simulink model "lineFollowerModel"  (R2020a)
settings: Solver=ode4  StartTime=0.0  StopTime=50  FixedStep=0.0001  RelTol=1e-3
values from neighbouring files (symbols this model uses):
  b = -0.05    [define_constants.m]
  cRoll = 0.1    [define_constants.m]
  g = 9.81    [define_constants.m]
  I_T = 0.1    [define_constants.m]
  I_yy = 5.0000e-05    (= 5e-05)    [define_constants.m]
  K = 0.0089    [define_constants.m]
  L = 2.3E-2    (= 0.023)    [define_constants.m]
  m_T = 1 * mass_scale    [define_constants.m]
  N = 50    [define_constants.m]
  R = 2.2    [define_constants.m]
  row1 = 0.1    [define_constants.m]
  row2 = row1*wheel_ratio_scale    [define_constants.m]
  sX_FL = 0.05    [define_constants.m]
  sX_FR = 0.05    [define_constants.m]
  sX_L = 0.05    [define_constants.m]
  sX_R = 0.05    [define_constants.m]
  sY_FL = 0.060    (= 0.06)    [define_constants.m]
  sY_FR = -0.060    (= -0.06)    [define_constants.m]
  sY_L = 0.03    [define_constants.m]
  sY_R = -0.03    [define_constants.m]
  Vmax = 12    [define_constants.m]
  W = line_width/2    [define_constants.m]
libraries: simulink x4
settings Model: Creator=Amir  LastModifiedBy=aekha
settings SFSimCC: CustomCodeUndefinedFunction=UseInterfaceOnly

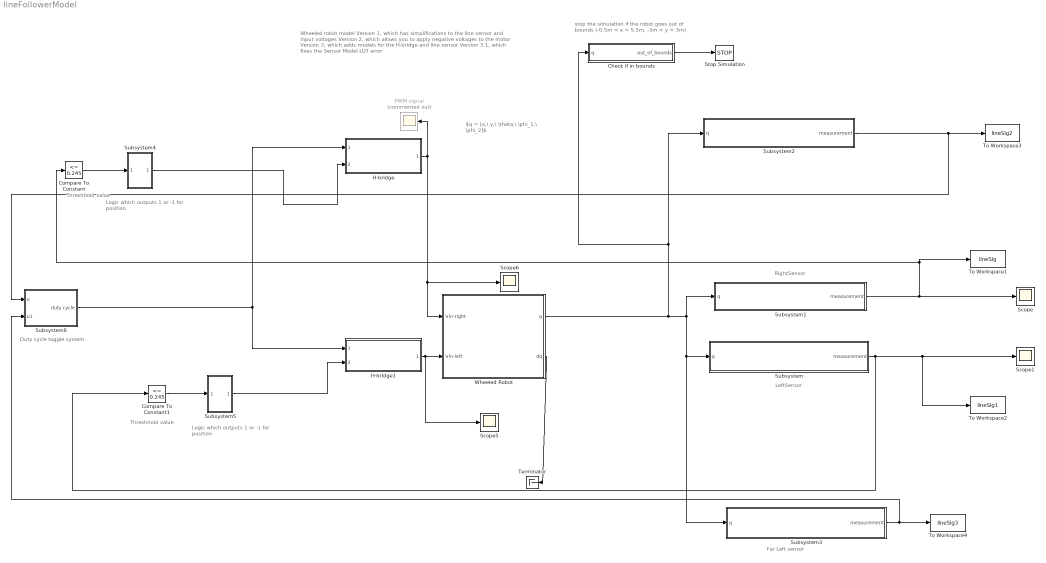
== system lineFollowerModel ==
  note: Threshhold value
  note: Duty cycle toggle system
  note: Far Left sensor
  note: Logic which outputs 1 or -1
      | for position
  note: LeftSensor
  note: RightSensor
  note: stop the simulation if the robot goes out of bounds (-0.5m < x < 5.5m, -3m < y < 3m)
  note: Wheeled robot model
      | Version 1, which has simplifications to the line sensor and input voltages
      | Version 2, which allows you to apply negative voltages to the motor
      | Version 3, which adds models for the H-bridge and line sensor
      | Version 3.1, which fixes the Sensor Model LUT error
  note: $q = [x,\ y,\ \theta,\ \phi_1,\ \phi_2]$
  note: Logic which outputs 1 or -1
      | for position
  note: Threshhold value
  Check if in bounds : MATLAB Function  TreatAsAtomicUnit=on
  Compare To Constant : simulink/Logic and Bit Operations/Compare To Constant  relop=<=  const=0.245  OutDataTypeStr=boolean
  Compare To Constant1 : simulink/Logic and Bit Operations/Compare To Constant  relop=<=  const=0.245  OutDataTypeStr=boolean
  H-bridge : Subsystem  ReferencedSubsystem=H_bridge
  H-bridge1 : Subsystem  ReferencedSubsystem=H_bridge
  PWM signal : Scope  Commented=on
  Scope{,1,5..6} (4 alike) : Scope
  Stop Simulation : Stop
  Subsystem : Subsystem
  Subsystem1 : Subsystem
  Subsystem2 : Subsystem
  Subsystem3 : Subsystem
  Subsystem4 : Subsystem
  Subsystem5 : Subsystem
  Subsystem6 : Subsystem
  Terminator : Terminator
  To Workspace1 : ToWorkspace  VariableName=lineSig  SampleTime=-1
  To Workspace2 : ToWorkspace  VariableName=lineSig1  SampleTime=-1
  To Workspace3 : ToWorkspace  VariableName=lineSig2  SampleTime=-1
  To Workspace4 : ToWorkspace  VariableName=lineSig3  SampleTime=-1
  Wheeled Robot : Subsystem
  wires:
  H-bridge/1 -> Scope6/1, Wheeled Robot/1(Vin-right), PWM signal/1
  H-bridge1/1 -> Scope5/1, Wheeled Robot/2(Vin-left)
  Wheeled Robot/2(dq) -> Terminator/1
  Check if in bounds/1(out_of_bounds) -> Stop Simulation/1
  Subsystem/1(measurement) -> Compare To Constant1/1, To Workspace2/1, Scope1/1
  Subsystem1/1(measurement) -> To Workspace1/1, Compare To Constant/1, Scope/1
  Subsystem3/1(measurement) -> Subsystem6/2(u1), To Workspace4/1
  Subsystem2/1(measurement) -> Subsystem6/1(u), To Workspace3/1
  Subsystem4/1(direction) -> H-bridge/2
  Wheeled Robot/1(q) -> Subsystem/1(q), Subsystem3/1(q), Subsystem1/1(q), Check if in bounds/1(q), Subsystem2/1(q)
  Subsystem5/1(direction) -> H-bridge1/2
  Compare To Constant/1 -> Subsystem4/1(In1)
  Compare To Constant1/1 -> Subsystem5/1(In1)
  Subsystem6/1(duty cycle) -> H-bridge1/1, H-bridge/1

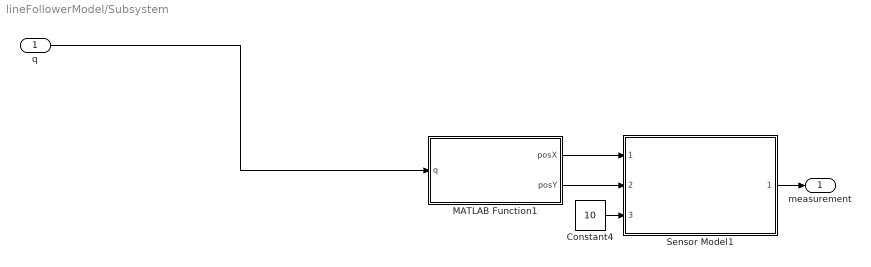
== system lineFollowerModel/Subsystem ==
  q : Inport
  Constant4 : Constant  Value=10
  MATLAB Function1 : MATLAB Function  TreatAsAtomicUnit=on
  Sensor Model1 : Subsystem  ReferencedSubsystem=Sensor_Model
  measurement : Outport
  wires:
  Constant4/1 -> Sensor Model1/3
  MATLAB Function1/2(posY) -> Sensor Model1/2
  Sensor Model1/1 -> measurement/1
  MATLAB Function1/1(posX) -> Sensor Model1/1
  q/1 -> MATLAB Function1/1(q)

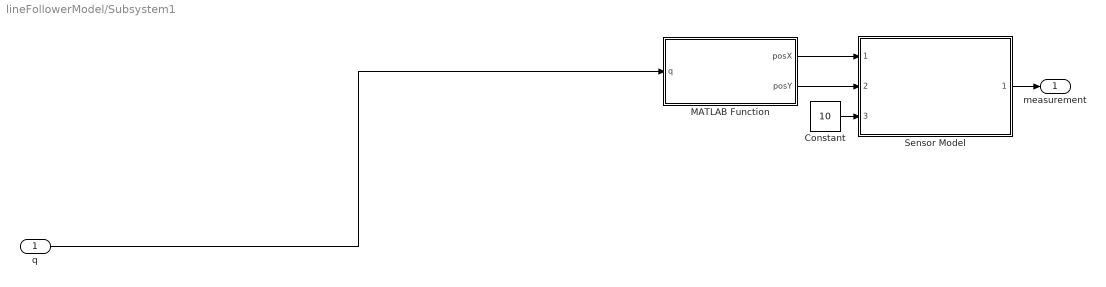
== system lineFollowerModel/Subsystem1 ==
  q : Inport
  Constant : Constant  Value=10
  MATLAB Function : MATLAB Function  TreatAsAtomicUnit=on
  Sensor Model : Subsystem  ReferencedSubsystem=Sensor_Model
  measurement : Outport
  wires:
  Constant/1 -> Sensor Model/3
  MATLAB Function/1(posX) -> Sensor Model/1
  q/1 -> MATLAB Function/1(q)
  Sensor Model/1 -> measurement/1
  MATLAB Function/2(posY) -> Sensor Model/2

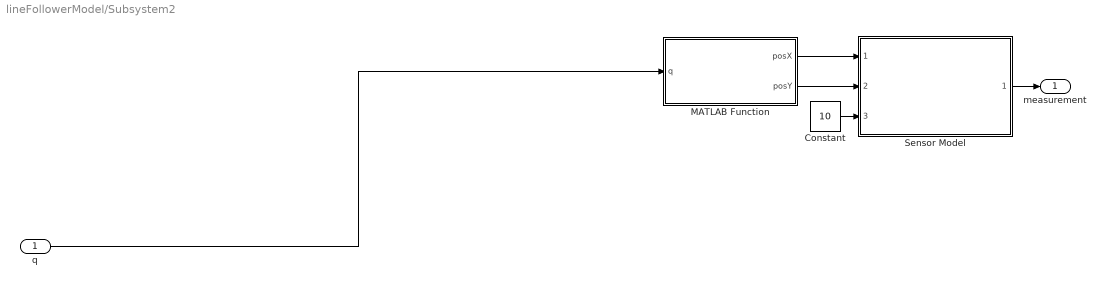
== system lineFollowerModel/Subsystem2 ==
  q : Inport
  Constant : Constant  Value=10
  MATLAB Function : MATLAB Function  TreatAsAtomicUnit=on
  Sensor Model : Subsystem  ReferencedSubsystem=Sensor_Model
  measurement : Outport
  wires:
  Constant/1 -> Sensor Model/3
  MATLAB Function/1(posX) -> Sensor Model/1
  q/1 -> MATLAB Function/1(q)
  Sensor Model/1 -> measurement/1
  MATLAB Function/2(posY) -> Sensor Model/2

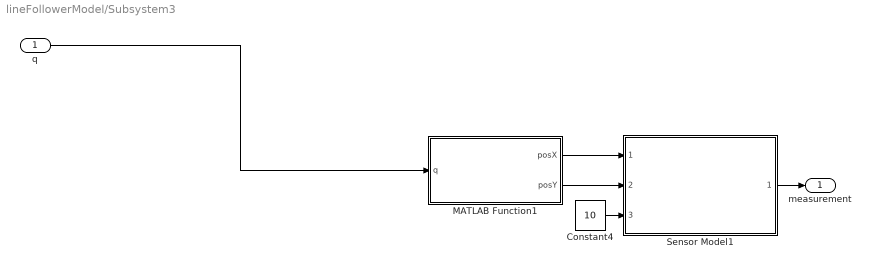
== system lineFollowerModel/Subsystem3 ==
  q : Inport
  Constant4 : Constant  Value=10
  MATLAB Function1 : MATLAB Function  TreatAsAtomicUnit=on
  Sensor Model1 : Subsystem  ReferencedSubsystem=Sensor_Model
  measurement : Outport
  wires:
  Constant4/1 -> Sensor Model1/3
  MATLAB Function1/2(posY) -> Sensor Model1/2
  Sensor Model1/1 -> measurement/1
  MATLAB Function1/1(posX) -> Sensor Model1/1
  q/1 -> MATLAB Function1/1(q)

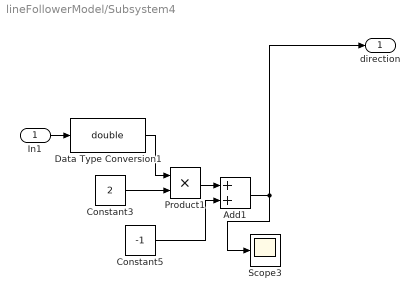
== system lineFollowerModel/Subsystem4 ==
  In1 : Inport
  Add1 : Sum
  Constant3 : Constant  Value=2
  Constant5 : Constant  Value=-1
  Data Type Conversion1 : DataTypeConversion  OutDataTypeStr=double
  Product1 : Product
  Scope3 : Scope
  direction : Outport
  wires:
  Data Type Conversion1/1 -> Product1/1
  Add1/1 -> direction/1, Scope3/1
  Constant5/1 -> Add1/2
  Product1/1 -> Add1/1
  In1/1 -> Data Type Conversion1/1
  Constant3/1 -> Product1/2

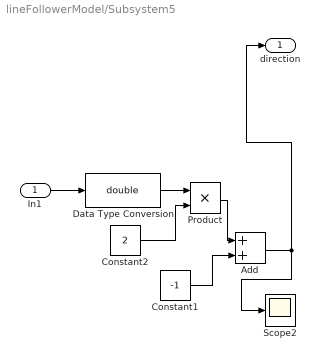
== system lineFollowerModel/Subsystem5 ==
  In1 : Inport
  Add : Sum
  Constant1 : Constant  Value=-1
  Constant2 : Constant  Value=2
  Data Type Conversion : DataTypeConversion  OutDataTypeStr=double
  Product : Product
  Scope2 : Scope
  direction : Outport
  wires:
  Constant2/1 -> Product/2
  Product/1 -> Add/1
  Add/1 -> direction/1, Scope2/1
  In1/1 -> Data Type Conversion/1
  Constant1/1 -> Add/2
  Data Type Conversion/1 -> Product/1

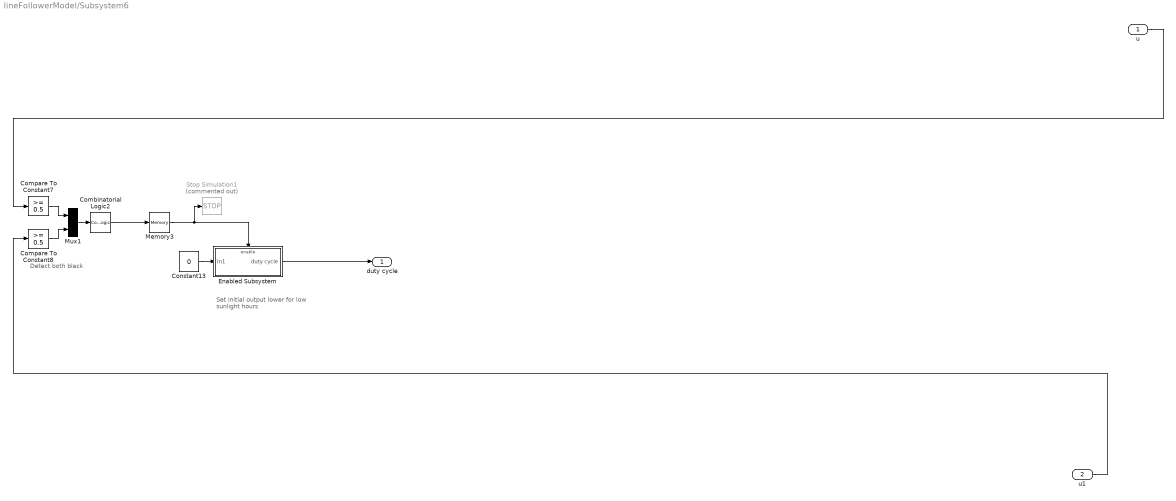
== system lineFollowerModel/Subsystem6 ==
  note: Detect both black
  note: Set initial output
      |  lower for low sunlight hours
  u : Inport
  u1 : Inport  Port=2
  Combinatorial Logic2 : CombinatorialLogic  TruthTable=[0;0;0;1]
  Compare To Constant7 : simulink/Logic and Bit Operations/Compare To Constant  relop=>=  const=0.5  OutDataTypeStr=boolean
  Compare To Constant8 : simulink/Logic and Bit Operations/Compare To Constant  relop=>=  const=0.5  OutDataTypeStr=boolean
  Constant13 : Constant  Value=0
  Enabled Subsystem : Subsystem  TreatAsAtomicUnit=on
  Memory3 : Memory
  Mux1 : Mux  Inputs=2
  Stop Simulation1 : Stop  Commented=on
  duty cycle : Outport
  wires:
  Compare To Constant8/1 -> Mux1/2
  Combinatorial Logic2/1 -> Memory3/1
  Memory3/1 -> Stop Simulation1/1, Enabled Subsystem/Enable
  Compare To Constant7/1 -> Mux1/1
  Mux1/1 -> Combinatorial Logic2/1
  Constant13/1 -> Enabled Subsystem/1(In1)
  u/1 -> Compare To Constant7/1
  Enabled Subsystem/1(duty cycle) -> duty cycle/1
  u1/1 -> Compare To Constant8/1

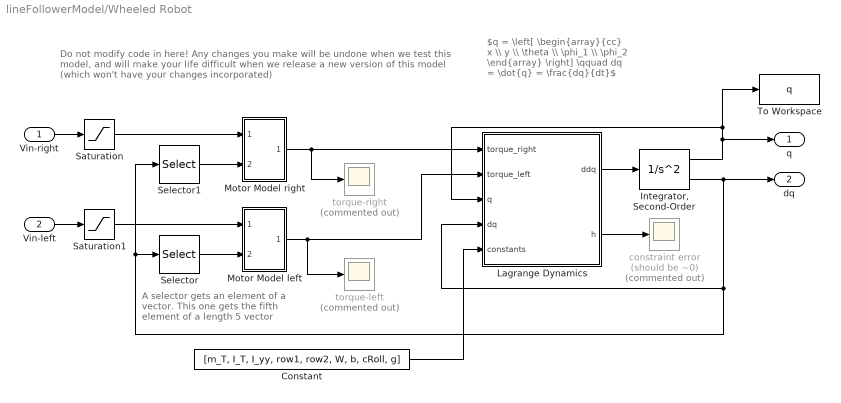
== system lineFollowerModel/Wheeled Robot ==
  note: A selector gets an element of a vector. This one gets the fifth element of a length 5 vector
  note: Do not modify code in here! Any changes you make will be undone when we test this model, and will make your life difficult when we release a new version of this model (which won't have your changes incorporated)
  note: $q = \left[ \begin{array}{cc} x \\ y \\ \theta \\ \phi_1 \\ \phi_2 \end{array} \right] \qquad dq = \dot{q} = \frac{dq}{dt}$
  Vin-right : Inport
  Vin-left : Inport  Port=2
  Constant : Constant  Value=[m_T, I_T, I_yy, row1, row2, W, b, cRoll, g]
  "Integrator, Second-Order" : SecondOrderIntegrator  ICX=[0 0 0 0 0]  ICDXDT=[0 0 0 0 0]
  Lagrange Dynamics : MATLAB Function  TreatAsAtomicUnit=on
  "Motor Model left " : Subsystem
  Motor Model right : Subsystem
  Saturation : Saturate  UpperLimit=Vmax  LowerLimit=-Vmax
  Saturation1 : Saturate  UpperLimit=Vmax  LowerLimit=-Vmax
  Selector : Selector  InputPortWidth=5  IndexOptions=Index vector (dialog)  Indices=[5]  OutputSizes=1
  Selector1 : Selector  InputPortWidth=5  IndexOptions=Index vector (dialog)  Indices=[4]  OutputSizes=1
  To Workspace : ToWorkspace  VariableName=q  SampleTime=0.01
  constraint error (should be ~0) : Scope  Commented=on
  torque-left : Scope  Commented=on
  torque-right : Scope  Commented=on
  q : Outport
  dq : Outport  Port=2
  wires:
  Selector/1 -> "Motor Model left "/2(Omega)
  Selector1/1 -> Motor Model right/2(Omega)
  Motor Model right/1(Tout) -> Lagrange Dynamics/1(torque_right), torque-right/1
  Vin-right/1 -> Saturation/1
  Vin-left/1 -> Saturation1/1
  "Integrator, Second-Order"/1 -> To Workspace/1, Lagrange Dynamics/3(q), q/1
  "Motor Model left "/1(Tout) -> Lagrange Dynamics/2(torque_left), torque-left/1
  "Integrator, Second-Order"/2 -> dq/1, Lagrange Dynamics/4(dq), Selector/1, Selector1/1
  Saturation/1 -> Motor Model right/1(Vin)
  Saturation1/1 -> "Motor Model left "/1(Vin)
  Lagrange Dynamics/1(ddq) -> "Integrator, Second-Order"/1
  Lagrange Dynamics/2(h) -> constraint error (should be ~0)/1
  Constant/1 -> Lagrange Dynamics/5(constants)

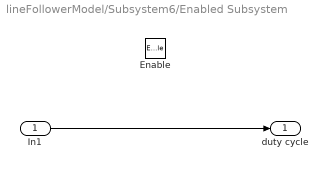
== system lineFollowerModel/Subsystem6/Enabled Subsystem ==
  In1 : Inport
  Enable : EnablePort
  duty cycle : Outport  InitialOutput=[0.2]
  wires:
  In1/1 -> duty cycle/1

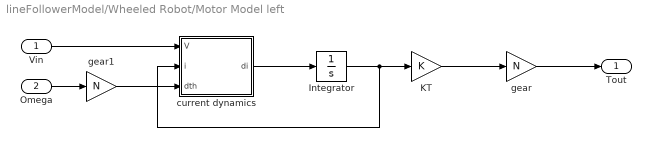
== system lineFollowerModel/Wheeled Robot/Motor Model left  ==
  Vin : Inport
  Omega : Inport  Port=2
  Integrator : Integrator
  KT : Gain  Gain=K
  current dynamics : MATLAB Function  TreatAsAtomicUnit=on
  gear : Gain  Gain=N
  gear1 : Gain  Gain=N
  Tout : Outport  VectorParamsAs1DForOutWhenUnconnected=off
  wires:
  gear1/1 -> current dynamics/3(dth)
  Integrator/1 -> current dynamics/2(i), KT/1
  Omega/1 -> gear1/1
  gear/1 -> Tout/1
  current dynamics/1(di) -> Integrator/1
  KT/1 -> gear/1
  Vin/1 -> current dynamics/1(V)

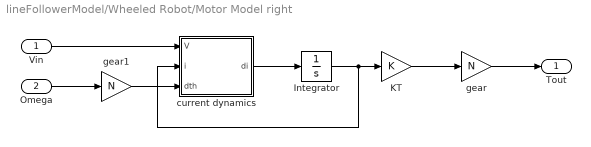
== system lineFollowerModel/Wheeled Robot/Motor Model right ==
  Vin : Inport
  Omega : Inport  Port=2
  Integrator : Integrator
  KT : Gain  Gain=K
  current dynamics : MATLAB Function  TreatAsAtomicUnit=on
  gear : Gain  Gain=N
  gear1 : Gain  Gain=N
  Tout : Outport  VectorParamsAs1DForOutWhenUnconnected=off
  wires:
  Vin/1 -> current dynamics/1(V)
  KT/1 -> gear/1
  current dynamics/1(di) -> Integrator/1
  gear/1 -> Tout/1
  Omega/1 -> gear1/1
  Integrator/1 -> current dynamics/2(i), KT/1
  gear1/1 -> current dynamics/3(dth)

== matlab function lineFollowerModel/Subsystem3/MATLAB Function1 ==
  data: posX output; q input; sY_FL parameter; sX_FL parameter; posY output
function [posX, posY] = sensorFarLeftPosition(q, sY_FL, sX_FL)

x = q(1);
y = q(2);
th = q(3);

% Position of sensor in inertial coordinates
% sX and sY are the sensor's X and Y offsets relative to the center of the
% line follow. By default, sX = 0.1m, sY = 0m. You can define sX and sY for
% each sensor on the robot
% You'll need to use a little geometry/math to calculate the position of
% the sensor in the world frame
posSens_I = [x + sX_FL*cos(th) - sY_FL*sin(th)
             y + sY_FL*cos(th) + sX_FL*sin(th)];

posX = posSens_I(1);
posY = posSens_I(2);

== matlab function lineFollowerModel/Wheeled Robot/Motor Model left /current dynamics ==
  data: V input; di output; i input; L parameter; K parameter; R parameter; dth input
function di = dyn(V, i, L, K, R, dth)

di = (V-K*dth-R*i)/L;

== matlab function lineFollowerModel/Wheeled Robot/Lagrange Dynamics ==
  settings: updateMethod=DISCRETE
  data: ddq output size=5; h output size=3; torque_right input; torque_left input; q input; dq input; constants input
%% These dynamics are based on: 
% https://robotics.caltech.edu/~me72/class/DiffDrive2.pdf
% Assume 'd' is 0
function [ddq, h] = dyn(torque_right, torque_left, q, dq, constants)
m_T = constants(1);
I_T = constants(2);
I_yy = constants(3);
row1 = constants(4);
row2 = constants(5);
W = constants(6);
b = constants(7);
cRoll = constants(8);
g = constants(9);

%% Admin
% x = q(1);
% y = q(2);
th = q(3);
% phi1 = q(4);
% phi2 = q(5);

dx = dq(1);
dy = dq(2);
dth = dq(3);
dphi1 = dq(4);
dphi2 = dq(5);


%% Calculate the matrices
% Mass
M = [m_T,   0,   0,    0,    0
       0, m_T,   0,    0,    0
       0,   0, I_T,    0,    0
       0,   0,   0, I_yy,    0
       0,   0,   0,    0, I_yy];

temp = [-sin(th), cos(th), cos(th)
         cos(th), sin(th), sin(th)
               0,     W/2,    -W/2
               0,  - row1,       0
               0,       0,   -row2];

C = transpose(temp);

temp = [ -dth*cos(th), -dth*sin(th), -dth*sin(th)
         -dth*sin(th),  dth*cos(th),  dth*cos(th)
                    0,            0,            0
                    0,            0,            0
                    0,            0,            0];

dC = transpose(temp);

% Input force
T = [0; 0; 0; torque_right + b*dphi1; torque_left + b*dphi2];

% Rolling resistance
vWheel1 = (W*dth)/2 + dx*cos(th) + dy*sin(th);
vWheel2 = dx*cos(th) - (W*dth)/2 + dy*sin(th);
sgnWheel1 = sign(vWheel1);
sgnWheel2 = sign(vWheel2);

F1 = -sgnWheel1*m_T*g*cRoll;
F2 = -sgnWheel2*m_T*g*cRoll;

% input force mapping
Q =  [F1*cos(th) + F2*cos(th)
      F1*sin(th) + F2*sin(th)
          (F1*W)/2 - (F2*W)/2
                            0
                            0];

%% Calculate Lagrange Multipliers
% lambda = -inv(C*inv(M)*transpose(C))*(C*inv(M)*(T+Q) + dC*dq);
lambda = -inv(C*(M\transpose(C)))*(C*(M\(T+Q)) + dC*dq);

h = [                          dy*cos(th) - dx*sin(th)
      (W*dth)/2 - dphi1*row1 + dx*cos(th) + dy*sin(th)
      dx*cos(th) - dphi2*row2 - (W*dth)/2 + dy*sin(th)];


%% Calculate acceleration
ddq = M\(transpose(C)*lambda + T + Q);

end

== matlab function lineFollowerModel/Wheeled Robot/Motor Model right/current dynamics ==
  data: V input; di output; i input; L parameter; K parameter; R parameter; dth input
function di = dyn(V, i, L, K, R, dth)

di = (V - K*dth - R*i)/L;

== matlab function lineFollowerModel/Subsystem1/MATLAB Function ==
  data: posX output; q input; sY_R parameter; sX_R parameter; posY output
function [posX, posY] = sensorRightPosition(q, sY_R, sX_R)

x = q(1);
y = q(2);
th = q(3);

% Position of sensor in inertial coordinates
% sX and sY are the sensor's X and Y offsets relative to the center of the
% line follow. By default, sX = 0.1m, sY = 0m. You can define sX and sY for
% each sensor on the robot
% You'll need to use a little geometry/math to calculate the position of
% the sensor in the world frame
posSens_I = [x + sX_R*cos(th) - sY_R*sin(th)
             y + sY_R*cos(th) + sX_R*sin(th)];

posX = posSens_I(1);
posY = posSens_I(2);

== matlab function lineFollowerModel/Subsystem/MATLAB Function1 ==
  data: posX output; q input; sY_L parameter; sX_L parameter; posY output
function [posX, posY] = sensorLeftPosition(q, sY_L, sX_L)

x = q(1);
y = q(2);
th = q(3);

% Position of sensor in inertial coordinates
% sX and sY are the sensor's X and Y offsets relative to the center of the
% line follow. By default, sX = 0.1m, sY = 0m. You can define sX and sY for
% each sensor on the robot
% You'll need to use a little geometry/math to calculate the position of
% the sensor in the world frame
posSens_I = [x + sX_L*cos(th) - sY_L*sin(th)
             y + sY_L*cos(th) + sX_L*sin(th)];

posX = posSens_I(1);
posY = posSens_I(2);

== matlab function lineFollowerModel/Check if in bounds ==
  data: q input; out_of_bounds output
function out_of_bounds = fcn(q)
x = q(1);
y = q(2);

in_bounds = -0.5 < x && x < 5.5 && -3 < y && y < 3;

out_of_bounds = ~in_bounds;

if out_of_bounds
    disp("Stopping simulation - robot is out of bounds!")
end

== matlab function lineFollowerModel/Subsystem2/MATLAB Function ==
  data: posX output; q input; sY_FR parameter; sX_FR parameter; posY output
function [posX, posY] = sensorFarRightPosition(q, sY_FR, sX_FR)

x = q(1);
y = q(2);
th = q(3);

% Position of sensor in inertial coordinates
% sX and sY are the sensor's X and Y offsets relative to the center of the
% line follow. By default, sX = 0.1m, sY = 0m. You can define sX and sY for
% each sensor on the robot
% You'll need to use a little geometry/math to calculate the position of
% the sensor in the world frame
posSens_I = [x + sX_FR*cos(th) - sY_FR*sin(th)
             y + sY_FR*cos(th) + sX_FR*sin(th)];

posX = posSens_I(1);
posY = posSens_I(2);
